simulink model "Vib_cal_model"  (R2019b)
settings: Solver=VariableStepAuto  StartTime=0.0  StopTime=0.02  RelTol=1e-3
settings Model: Creator=YANG  LastModifiedBy=YANG

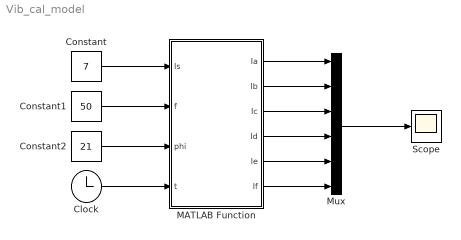
== system Vib_cal_model ==
  Clock : Clock
      settings: Decimation=1000
  Constant : Constant  Value=7
  Constant1 : Constant  Value=50
  Constant2 : Constant  Value=21
  MATLAB Function : MATLAB Function  TreatAsAtomicUnit=on
  Mux : Mux  Inputs=6
  Scope : Scope
  wires:
  Constant/1 -> MATLAB Function/1(Is)
  Constant1/1 -> MATLAB Function/2(f)
  Constant2/1 -> MATLAB Function/3(phi)
  MATLAB Function/1(Ia) -> Mux/1
  MATLAB Function/2(Ib) -> Mux/2
  MATLAB Function/3(Ic) -> Mux/3
  MATLAB Function/4(Id) -> Mux/4
  MATLAB Function/5(Ie) -> Mux/5
  MATLAB Function/6(If) -> Mux/6
  Mux/1 -> Scope/1
  Clock/1 -> MATLAB Function/4(t)

== matlab function Vib_cal_model/MATLAB Function ==
  data: Is input; Ia output; f input; phi input; Ib output; Ic output; Id output; Ie output; If output; t input
function [Ia,Ib,Ic,Id,Ie,If] = fcn(Is,f,phi,t)
Ia=Is*sin(2*pi*f*t+phi*pi/180);
Ib=Is*sin(2*pi*f*t+phi*pi/180-2*pi/3);
Ic=Is*sin(2*pi*f*t+phi*pi/180+2*pi/3);
Id=Is*sin(2*pi*f*t+phi*pi/180-pi/6);
Ie=Is*sin(2*pi*f*t+phi*pi/180-pi/6-2*pi/3);
If=Is*sin(2*pi*f*t+phi*pi/180-pi/6+2*pi/3);
end
